simulink model "Generic_13"  (R2022b)
settings: Solver=VariableStepAuto  StartTime=0.0  StopTime=10.0  RelTol=1e-3
values from neighbouring files (symbols this model uses):
  A = cell2mat(A_cell)    [MPCController1.m]    (also in MPC_Fmincon.m)
  B = cell2mat(B_cell)    [MPCController1.m]    (also in MPC_Fmincon.m)
  brake_select = ones(length(speed), length(steering_angle))    [TwoDLook_uptable.m]
  curvature = 0.000:0.001:1    [TwoDLook_uptable.m]
  m = 1600    [MPCController1.m]    (also in MPCController2.m; MPC_Fmincon.m)
  speed = 0:0.1:100    [TwoDLook_uptable.m]
undefined symbols (not defined in the file or in its folder): Amplifier, DiscIntNeverNeededParam, K_d_yawrate, K_dsteering, k_speed, k_stanley, kd, ki, kp, path_curvature
libraries: CarMaker4SL x121, simulink x12, cstblocks x7, autolibshared x1, mpcadaslib x1
(part 5 of 5)

== matlab function Generic_13/CreateBus VhclCtrl/Subsystem/MATLAB Function ==
  data: currentPosition input; currentHeading output; nextWaypoint input; desiredHeading output; headingError output
function [currentHeading, desiredHeading, headingError] = calculateHeadingError(currentPosition, nextWaypoint)
    % Calculate current heading, desired heading, and heading error for Stanley controller
    % Inputs:
    %   - currentPosition: Current position of the vehicle [x, y] (single points)
    %   - nextWaypoint: Next waypoint on the path [x, y]
    % Outputs:
    %   - currentHeading: Current heading of the vehicle (in radians)
    %   - desiredHeading: Desired heading or reference angle (in radians)
    %   - headingError: Heading error (in radians)
    function angle = wrapToPi(angle)
    % Wrap angle to the range [-pi, pi]
    angle = mod(angle + pi, 2 * pi) - pi;
    end
    % Extract x and y coordinates from the current position
    x = currentPosition(1);
    y = currentPosition(2);
    
    % Calculate the vector from the vehicle to the next waypoint
    headingVector = nextWaypoint - [x, y];

    % Calculate the current heading
    currentHeading = atan2(headingVector(2), headingVector(1));
    disp(currentHeading)
    disp('next')
    % Calculate the desired heading (heading of the vector between the current position and next waypoint)
    desiredHeading = atan2(nextWaypoint(2) - y, nextWaypoint(1) - x);
    disp(desiredHeading)
    % Calculate heading error
    headingError = wrapToPi(desiredHeading - currentHeading);
end

== matlab function Generic_13/CreateBus VhclCtrl/Stanley  steering & speed//Brake controller/Stanley controller with path_planning/Stanley controller with path_planning/MATLAB Function ==
  data: path input; dev input; e output; yaw input; speed_act input; err_fr_axle output; cross_track_steering output; heading_err output; steering output
function [e, err_fr_axle, cross_track_steering, heading_err, steering]  = conversion(path,dev,yaw,speed_act)
%path = [path_x;path_y];
function distance = calc_distance(pt,v1,v2)
    vect = v1 - v2;
    p_to_vect = pt - v2;
    crossVP = cross(vect,p_to_vect);
    distance = norm(crossVP) / norm(vect) * crossVP(3)/abs(crossVP(3));
end

e = zeros(1);
cross_track_steering = zeros(1);
heading_err = zeros(1);
steering=zeros(1);
err_fr_axle = zeros(1);

k_exp = 1.3059;
k = 15.028 + speed_act^k_exp;
k_ref = 2.62;

% path_index = fix(k_path * speed_act);
% if path_index > 13
%     path_index = 13;
% end
% 
% P_prev = path(:,6 + path_index);
% P_next = path(:,7 + path_index);

fr_axle = [-1.488 0 0];
distances = sqrt((path(1,:) - 1.488).^2 + (path(2,:) - 0).^2);
% Find the index of the closest point on the path
[~,err_fr_axle_ind] = min(distances);
if err_fr_axle_ind == 1
    err_fr_axle_ind = 2;
end
err_fr_axle = calc_distance(fr_axle,[path(1,err_fr_axle_ind - 1) path(2,err_fr_axle_ind - 1) 0],[path(1,err_fr_axle_ind) path(2,err_fr_axle_ind) 0]);

B = [-1.488 + k_ref * (speed_act / 27) 0 0];
distances_err = sqrt((path(1,:) - B(1)).^2 + (path(2,:) - 0).^2);
[~,err_ind] = min(distances_err);
if err_ind < 2
    err_ind = 2;
end
error = calc_distance(B,[path(1,err_ind - 1) path(2,err_ind - 1) 0],[path(1,err_ind) path(2,err_ind) 0]);


P_prev = path(:, err_ind-1);
P_next = path(:, err_ind);

x1 = P_prev(1,1);
y1 = P_prev(2,1);
x2 = P_next(1,1);
y2 = P_next(2,1);

a = (y2 - y1)/-(x2 + x1);
b = 1;
%c = -x1 * (y2 - y1) + y1 * (x2 - x1);


if speed_act ~= 0
    %e = c+b*y1/sqrt((a^2)+(b^2));
    e = error;
    
    cross_track_steering = atan(k * e / speed_act);
    heading_err = atan(-a / b) - yaw;
    %heading_err = 1/(tan(-a/b))-yaw;
    steering = heading_err + cross_track_steering;
end
end
